simulink model "exemplo_bloco_Main"  (R2015a)
settings: Solver=ode45  StartTime=0.0  StopTime=10  RelTol=1e-6
settings Model: CovSFcnEnable=off  Creator=Mauricio  LastModifiedBy=YecidMoreno
settings DebuggingCC: SolverPrmCheckMsg=warning

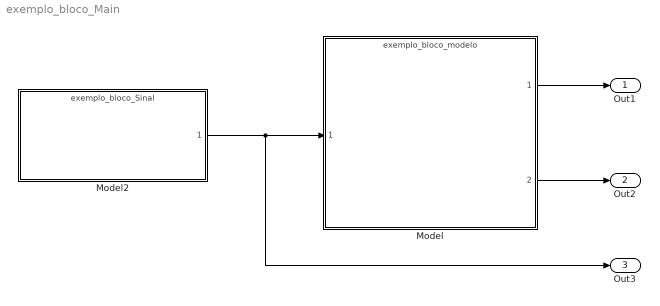
== system exemplo_bloco_Main ==
  Model : ModelReference  ModelNameDialog=exemplo_bloco_modelo.slx  SimulationMode=Normal  ModelReferenceVersion=1.117  CopyOfModelName=exemplo_bloco_modelo.slx  DefaultDataLogging=on
  Model2 : ModelReference  ModelNameDialog=exemplo_bloco_Sinal.slx  SimulationMode=Normal  ModelReferenceVersion=1.12  CopyOfModelName=exemplo_bloco_Sinal.slx  DefaultDataLogging=on
  Out1 : Outport
  Out2 : Outport  Port=2
  Out3 : Outport  Port=3
  wires:
  Model/2 -> Out2/1
  Model/1 -> Out1/1
  Model2/1 -> Out3/1, Model/1
